simulink model "ms_project_cleaned_from_autosave"  (R2020b)
settings: Solver=VariableStepAuto  StartTime=0.0  StopTime=2  RelTol=1e-3
libraries: powerlib x19, simulink x7, powerlib_meascontrol x6, fillib x2, re_lib x1
settings Model: Creator=mcapuano  LastModifiedBy=mcapuano

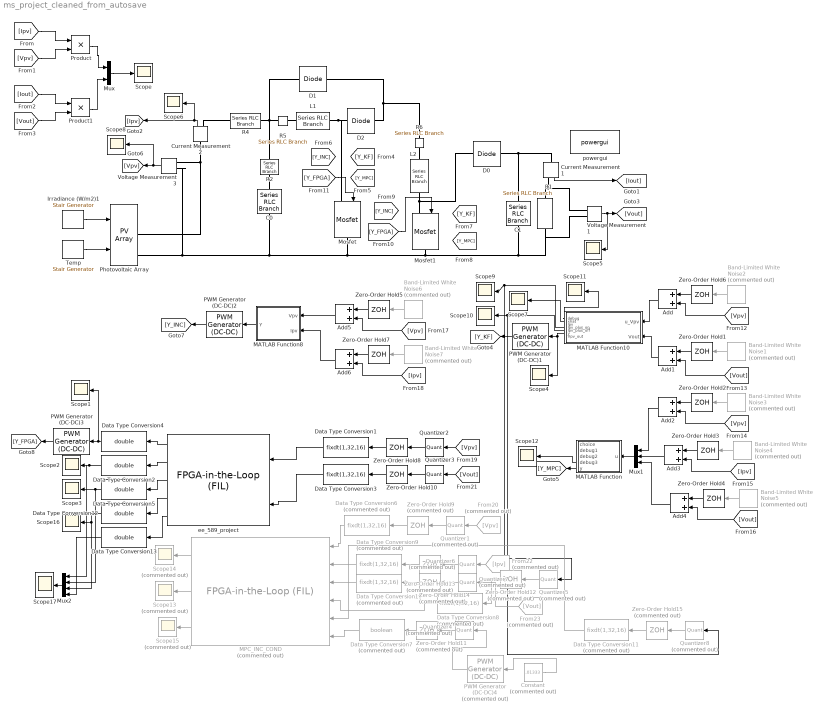
== system ms_project_cleaned_from_autosave ==
  " Temp" : powerlib_meascontrol/Pulse & Signal Generators/Stair Generator  t=[0 .5 1 1.5]  e=[25 25 35 45]  Ts=15e-6
  Add{,1..6} (7 alike) : Sum
  Band-Limited White Noise{1..7} (7 alike) : simulink/Sources/Band-Limited White Noise  Commented=on  Cov=[.00001]  Ts=15e-6  seed=[23341]
  C0 : powerlib/Elements/Series RLC Branch  LConnTagsString=__new0  RConnTagsString=__new0  BranchType=C  Resistance=1e-4  Inductance=200e-6  SetiL0=off  InitialCurrent=0  Capacitance=260e-6  Setx0=on  InitialVoltage=0  Measurements=None
  C1 : powerlib/Elements/Series RLC Branch  LConnTagsString=__new0  RConnTagsString=__new0  BranchType=C  Resistance=1e-4  Inductance=200e-6  SetiL0=off  InitialCurrent=0  Capacitance=260e-6  Setx0=on  InitialVoltage=0  Measurements=None
  Constant : Constant  Commented=on  Value=.01333
  Current Measurement1 : powerlib/Measurements/Current Measurement  PhasorSimulation=off  OutputType=Complex  PSBequivalent=0
  Current Measurement2 : powerlib/Measurements/Current Measurement  PhasorSimulation=off  OutputType=Complex  PSBequivalent=0
  D0 : powerlib/Power Electronics/Diode  Ron=1e-3  Lon=0  Vf=0  IC=0  UseSnubber=off  Rs=inf  Cs=inf  Measurements=off
  D1 : powerlib/Power Electronics/Diode  Ron=1e-3  Lon=0  Vf=0  IC=0  UseSnubber=off  Rs=inf  Cs=inf  Measurements=off
  D2 : powerlib/Power Electronics/Diode  Ron=1e-3  Lon=0  Vf=0  IC=0  UseSnubber=off  Rs=inf  Cs=inf  Measurements=off
  Data Type Conversion1 : DataTypeConversion  OutDataTypeStr=fixdt(1,32,16)
  Data Type Conversion{6,8..11} (5 alike) : DataTypeConversion  Commented=on  OutDataTypeStr=fixdt(1,32,16)
  Data Type Conversion{2,4..5,12..13} (5 alike) : DataTypeConversion  OutDataTypeStr=double
  Data Type Conversion3 : DataTypeConversion  OutDataTypeStr=fixdt(1,32,16)
  Data Type Conversion7 : DataTypeConversion  Commented=on  OutDataTypeStr=boolean
  From20 : From  Commented=on  GotoTag=Vpv
  From22 : From  Commented=on  GotoTag=Ipv
  From23 : From  Commented=on  GotoTag=Vout
  Irradiance (W/m2)1 : powerlib_meascontrol/Pulse & Signal Generators/Stair Generator  t=[0 .5]  e=[800 1000]  Ts=15e-6
  L1 : powerlib/Elements/Series RLC Branch  LConnTagsString=__new0  RConnTagsString=__new0  BranchType=L  Resistance=1e-4  Inductance=3e-3  SetiL0=on  InitialCurrent=0  Capacitance=30e-6  Setx0=off  InitialVoltage=150  Measurements=None
  L2 : powerlib/Elements/Series RLC Branch  LConnTagsString=__new0  RConnTagsString=__new0  BranchType=L  Resistance=1e-4  Inductance=3e-3  SetiL0=on  InitialCurrent=0  Capacitance=30e-6  Setx0=off  InitialVoltage=150  Measurements=None
  MATLAB Function : MATLAB Function  TreatAsAtomicUnit=on  SystemSampleTime=15e-6
  MATLAB Function10 : MATLAB Function  TreatAsAtomicUnit=on  SystemSampleTime=15e-6
  MATLAB Function8 : MATLAB Function  TreatAsAtomicUnit=on  SystemSampleTime=15e-6
  MPC_INC_COND : fillib/FPGA-in-the-Loop (FIL)  Commented=on  ForceInterfaceUpdate=0.67874
      settings: SourceProductBaseCode=ES,HD
  Mosfet : powerlib/Power Electronics/Mosfet  Ron=1e-3  Lon=0  Rd=1e-3  Vfd=0  IC=0  Rs=1e6  Cs=inf  Measurements=off
  Mosfet1 : powerlib/Power Electronics/Mosfet  Ron=1e-3  Lon=0  Rd=1e-3  Vfd=0  IC=0  Rs=1e6  Cs=inf  Measurements=off
  Mux : Mux  Inputs=2
  Mux1 : Mux  Inputs=3
  Mux2 : Mux
  PWM Generator (DC-DC)1 : powerlib_meascontrol/Pulse & Signal Generators/PWM Generator (DC-DC)  Fsw=66.67e3  Ts=0
  PWM Generator (DC-DC)2 : powerlib_meascontrol/Pulse & Signal Generators/PWM Generator (DC-DC)  Fsw=66.67e3  Ts=0
  PWM Generator (DC-DC)3 : powerlib_meascontrol/Pulse & Signal Generators/PWM Generator (DC-DC)  Fsw=66.67e3  Ts=0
  PWM Generator (DC-DC)4 : powerlib_meascontrol/Pulse & Signal Generators/PWM Generator (DC-DC)  Commented=on  Fsw=66.67e3  Ts=0
  Photovoltaic Array : re_lib/Solar/PV Array  Npar=1  Nser=1  PlotType=array @ 25 deg.C & specified irradiances  S_vec=[600 800 1000 1200]  Temp_C_vec=[25 50 75 100]  ModuleName=Kyocera Solar KC200GT  PlotWhenSelected=off  Pm=200.143  Ncell=54  Voc=32.9  Isc=8.21  Vm=26.3  Im=7.61  beta_Voc_pc=-0.355  alpha_Isc_pc=0.06  beta_Voc=-0.11679  alpha_Isc=0.004926  IL=8.2288  I0=2.3234e-10  nI=0.97734  Rsh=150.6844  Rs=0.34484  RobustModel=off  RobustCellTemperature=313.3991  BAL=on  Tc=1e-6  Tfilter=5e-5
      settings: AttributesFormatString=|
      | %<ModuleName>
      | %<Nser>-module string
      | %<Npar> parallel strings
  Product : Product
  Product1 : Product
  Quantizer{1,4..8} (6 alike) : Quantizer  Commented=on  QuantizationInterval=15e-6
  Quantizer2 : Quantizer  QuantizationInterval=15e-6
  Quantizer3 : Quantizer  QuantizationInterval=15e-6
  R1 : powerlib/Elements/Series RLC Branch  LConnTagsString=__new0  RConnTagsString=__new0  BranchType=R  Resistance=100  Inductance=200e-6  SetiL0=off  InitialCurrent=0  Capacitance=400e-6  Setx0=off  InitialVoltage=0  Measurements=None
  R2 : powerlib/Elements/Series RLC Branch  LConnTagsString=__new0  RConnTagsString=__new0  BranchType=R  Resistance=.01  Inductance=200e-6  SetiL0=off  InitialCurrent=0  Capacitance=400e-6  Setx0=off  InitialVoltage=0  Measurements=None
  R4 : powerlib/Elements/Series RLC Branch  LConnTagsString=__new0  RConnTagsString=__new0  BranchType=R  Resistance=1  Inductance=200e-6  SetiL0=off  InitialCurrent=0  Capacitance=400e-6  Setx0=off  InitialVoltage=0  Measurements=None
  R5 : powerlib/Elements/Series RLC Branch  LConnTagsString=__new0  RConnTagsString=__new0  BranchType=R  Resistance=1  Inductance=200e-6  SetiL0=off  InitialCurrent=0  Capacitance=400e-6  Setx0=off  InitialVoltage=0  Measurements=None
  R6 : powerlib/Elements/Series RLC Branch  LConnTagsString=__new0  RConnTagsString=__new0  BranchType=R  Resistance=1  Inductance=200e-6  SetiL0=off  InitialCurrent=0  Capacitance=400e-6  Setx0=off  InitialVoltage=0  Measurements=None
  Scope{,1..12,16..17} (15 alike) : Scope
  Scope13 : Scope  Commented=on
  Scope14 : Scope  Commented=on
  Scope15 : Scope  Commented=on
  Voltage Measurement1 : powerlib/Measurements/Voltage Measurement  PhasorSimulation=off  OutputType=Complex  PSBequivalent=0
  Voltage Measurement3 : powerlib/Measurements/Voltage Measurement  PhasorSimulation=off  OutputType=Complex  PSBequivalent=0
  Zero-Order Hold{1..7} (7 alike) : ZeroOrderHold  SampleTime=15e-6
  Zero-Order Hold10 : ZeroOrderHold  SampleTime=200e-9
  Zero-Order Hold{9,11..15} (6 alike) : ZeroOrderHold  Commented=on  SampleTime=200e-9
  Zero-Order Hold8 : ZeroOrderHold  SampleTime=200e-9
  ee_589_project : fillib/FPGA-in-the-Loop (FIL)  ForceInterfaceUpdate=0.046171
      settings: SourceProductBaseCode=ES,HD
  powergui : powerlib/powergui  Priority=1  SimulationMode=Continuous  SampleTime=50e-6  frequency=60  Iterations=50  frequencyindice=0  Pbase=100e6  ErrMax=1e-4  UnitsV=kV  UnitsW=MW  buscounter=0  FunctionMessages=off  echomessages=off  EnableUseOfTLC=off  CurrentSourceSwitches=off  DisableSnubberDevices=off  DisableRonSwitches=off  DisableVfSwitches=off  DisplayEquations=off  AutomaticDiscreteSolvers=off  SolverType=Tustin/Backward Euler (TBE)  Interpol=off  ExternalGateDelay=off  methode=off  Ts=100  x0status=blocks  SPID=on  SwTol=0  HookPort=off  NonlinearTolerance=1e-4  nMaxIteration=100  ContinueOnMaxIteration=off  RestoreLinks=warning  ResistiveCurrentMeasurement=off  Frange=[0:2:500]  Ylog=off  Xlog=on  ShowGrid=off  save=off  variable=ZData  structure=0  ZoomFFT=off  StartTime=0.0  cycles=1  DisplayStyle=1  fundamental=60  FreqAxis=off  MaxFrequency=1000  frequencyindicesteady=1  RmsSteady=1  display=off
  wires:
  Irradiance (W/m2)1/1 -> Photovoltaic Array/1
  " Temp"/1 -> Photovoltaic Array/2
  Voltage Measurement3/1 -> Scope8/1, [Vpv]
  Current Measurement2/1 -> Scope6/1, [Ipv]
  Voltage Measurement1/1 -> Scope5/1, [Vout]
  Current Measurement1/1 -> [Iout]
  [Ipv] -> Product/1
  [Vpv] -> Product/2
  Mux/1 -> Scope/1
  Product/1 -> Mux/1
  [Vout] -> Product1/2
  [Iout] -> Product1/1
  Product1/1 -> Mux/2
  Band-Limited White Noise2/1 -> Zero-Order Hold6/1
  MATLAB Function10/6(y) -> Scope4/1, PWM Generator (DC-DC)1/1
  PWM Generator (DC-DC)1/1 -> [Y_KF]
  Add/1 -> MATLAB Function10/1(u_Vpv)
  Zero-Order Hold6/1 -> Add/1
  Band-Limited White Noise1/1 -> Zero-Order Hold1/1
  Zero-Order Hold1/1 -> Add1/1
  Add1/1 -> MATLAB Function10/2(Vout)
  [Vpv] -> Add/2
  [Vout] -> Add1/2
  MATLAB Function/5(y) -> [Y_MPC]
  Mux1/1 -> MATLAB Function/1(u)
  [Vpv] -> Add2/2
  Band-Limited White Noise3/1 -> Zero-Order Hold2/1
  Zero-Order Hold2/1 -> Add2/1
  Add2/1 -> Mux1/1
  [Ipv] -> Add3/2
  Band-Limited White Noise4/1 -> Zero-Order Hold3/1
  Zero-Order Hold3/1 -> Add3/1
  Add3/1 -> Mux1/2
  Band-Limited White Noise5/1 -> Zero-Order Hold4/1
  [Vout] -> Add4/2
  Zero-Order Hold4/1 -> Add4/1
  Add4/1 -> Mux1/3
  [Vpv] -> Add5/2
  Band-Limited White Noise7/1 -> Zero-Order Hold7/1
  Band-Limited White Noise6/1 -> Zero-Order Hold5/1
  [Ipv] -> Add6/2
  Zero-Order Hold7/1 -> Add6/1
  Zero-Order Hold5/1 -> Add5/1
  Add5/1 -> MATLAB Function8/1(Vpv)
  Add6/1 -> MATLAB Function8/2(Ipv)
  [Vpv] -> Quantizer2/1
  Quantizer2/1 -> Zero-Order Hold8/1
  Zero-Order Hold8/1 -> Data Type Conversion1/1
  Quantizer3/1 -> Zero-Order Hold10/1
  Zero-Order Hold10/1 -> Data Type Conversion3/1
  Data Type Conversion3/1 -> ee_589_project/2
  [Vout] -> Quantizer3/1
  ee_589_project/1 -> Data Type Conversion4/1
  PWM Generator (DC-DC)2/1 -> [Y_INC]
  MATLAB Function8/1(Y) -> PWM Generator (DC-DC)2/1
  PWM Generator (DC-DC)3/1 -> [Y_FPGA]
  Data Type Conversion4/1 -> Scope1/1, PWM Generator (DC-DC)3/1
  Data Type Conversion1/1 -> ee_589_project/1
  ee_589_project/2 -> Data Type Conversion2/1
  ee_589_project/3 -> Data Type Conversion5/1
  Data Type Conversion2/1 -> Mux2/1, Scope2/1
  Data Type Conversion5/1 -> Mux2/2, Scope3/1
  MATLAB Function10/2(xhat) -> Scope7/1
  MATLAB Function10/4(Ipv_plus_on) -> Quantizer5/1, Scope9/1
  MATLAB Function10/5(Ipv_plus_off) -> Quantizer8/1, Scope10/1
  MATLAB Function10/1(debug) -> Scope11/1
  MATLAB Function/4(debug3) -> Scope12/1
  Data Type Conversion6/1 -> MPC_INC_COND/1
  Zero-Order Hold9/1 -> Data Type Conversion6/1
  Quantizer1/1 -> Zero-Order Hold9/1
  From20/1 -> Quantizer1/1
  Zero-Order Hold12/1 -> Data Type Conversion8/1
  Quantizer5/1 -> Zero-Order Hold12/1
  Data Type Conversion8/1 -> MPC_INC_COND/4
  Zero-Order Hold13/1 -> Data Type Conversion9/1
  Quantizer6/1 -> Zero-Order Hold13/1
  Data Type Conversion9/1 -> MPC_INC_COND/2
  Zero-Order Hold14/1 -> Data Type Conversion10/1
  Quantizer7/1 -> Zero-Order Hold14/1
  Data Type Conversion10/1 -> MPC_INC_COND/3
  From22/1 -> Quantizer6/1
  From23/1 -> Quantizer7/1
  MPC_INC_COND/3 -> Scope15/1
  MPC_INC_COND/1 -> Scope14/1
  MPC_INC_COND/2 -> Scope13/1
  Data Type Conversion11/1 -> MPC_INC_COND/5
  Zero-Order Hold15/1 -> Data Type Conversion11/1
  Quantizer8/1 -> Zero-Order Hold15/1
  Data Type Conversion7/1 -> MPC_INC_COND/6
  Zero-Order Hold11/1 -> Data Type Conversion7/1
  Quantizer4/1 -> Zero-Order Hold11/1
  PWM Generator (DC-DC)4/1 -> Quantizer4/1
  Constant/1 -> PWM Generator (DC-DC)4/1
  [Y_FPGA] -> Mosfet/1
  [Y_FPGA] -> Mosfet1/1
  ee_589_project/4 -> Data Type Conversion12/1
  ee_589_project/5 -> Data Type Conversion13/1
  Data Type Conversion12/1 -> Mux2/3, Scope16/1
  Mux2/1 -> Scope17/1
  Data Type Conversion13/1 -> Mux2/4
  connections:
  Voltage Measurement3/LConn1 -- Current Measurement2/LConn1 -- Photovoltaic Array/RConn1
  R4/LConn1 -- Current Measurement2/RConn1
  R5/LConn1 -- R4/RConn1 -- R2/LConn1 -- D1/LConn1
  R5/RConn1 -- L1/LConn1
  D2/LConn1 -- Mosfet/LConn1 -- L1/RConn1
  D1/RConn1 -- R6/LConn1 -- D2/RConn1
  L2/LConn1 -- R6/RConn1
  Mosfet1/LConn1 -- D0/LConn1 -- L2/RConn1
  C0/LConn1 -- R2/RConn1
  C0/RConn1 -- Voltage Measurement3/LConn2 -- Photovoltaic Array/RConn2 -- Voltage Measurement1/LConn2 -- R1/RConn1 -- C1/RConn1 -- Mosfet1/RConn1 -- Mosfet/RConn1
  C1/LConn1 -- Current Measurement1/LConn1 -- D0/RConn1
  Current Measurement1/RConn1 -- Voltage Measurement1/LConn1 -- R1/LConn1

== matlab function ms_project_cleaned_from_autosave/MATLAB Function ==
  settings: updateMethod=DISCRETE
  data: choice output; debug1 output; debug2 output; debug3 output; u input; y output
function [choice, debug1, debug2,debug3, y]= fcn(u)
Vpv=u(1);
Ipv=u(2);
Vout=u(3);

%This module contains the MPC-MPPT Control Algorithm

%The MPC module follows the flow chart of Fig. 8 in Referenced Research Paper

%This MATLAB fn block's settings have been changed to have a sampling rate
%of 15uS instead of being continous sample mode


%prevent crazy simulation transients from breaking the algorithm:
if (Ipv > 10)
    Ipv = 1;
end

persistent Vpv_t_1; %previous Vpv Sample
if isempty(Vpv_t_1)
    Vpv_t_1 = 0;
end
persistent Ipv_t_1; %previous Ipv Sample
if isempty(Ipv_t_1)
    Ipv_t_1 = 0;
end
persistent Dpv_t_1; % Iref (output) value from what is now 2 timesteps ago
if isempty(Dpv_t_1)
    Dpv_t_1 = 0;
end
persistent Dpv;  %Previous / Most recent Iref (output) Calc
if isempty(Dpv)
    Dpv = 0;
end

Ts = 15e-6; %sample rate
L = 3e-3; %inductance

Power = Vpv * Ipv;
delta_P = Power - (Vpv_t_1 * Ipv_t_1);
delta_V = Vpv - Vpv_t_1;
delta_I = Ipv - Ipv_t_1;
delta_D = Dpv - Dpv_t_1;


%fixed vs adaptive
S = .001;
M = 10;
Z =.001;%delta_P/delta_V * exp(-M*Dpv); %.0005; %fixed 
%Z = scale_factor_C * abs(delta_I * delta_D); %adaptive

% custom adaptive to fix issues with no change causing 0 step size
 %adapZ = scale_factor_C * abs(delta_I * delta_D);
% if(adapZ > .1)
%     Z = .1;
% elseif(adapZ > .001)
%     Z = adapZ;
% else
%     Z = .001;
% end


Ipred_1 = Ipv + 2*(Ts/L) * Vpv; %MPC prediction for switch = 1
Ipred_0 = Ipv + (Ts/(2*L)* (Vpv - Vout)); %MPC prediction for switch = 0 

if delta_V == 0 %Inc. Cond. Algo to determin Iref
    if delta_I == 0 
        Iref = Dpv; choice = 0;
    else
        if delta_I > 0
            Iref = Dpv - Z; choice = 1;
        else
            Iref = Dpv + Z; choice = 2;
        end
    end
else
    if (Ipv + (delta_I/delta_V) * Vpv) == 0
        Iref = Dpv; choice = 3;
    else
        if (Ipv + (delta_I/delta_V) * Vpv) > 0
            Iref = Dpv - Z; choice = 4;
        else
            Iref = Dpv + Z; choice = 5;
        end
    end
end

G1 = abs(Iref - Ipred_1); %Optimize MPC by applying Iref
G0 = abs(Iref - Ipred_0);
if G1 < G0
    y = 1;
else
    y = 0;
end

if (Iref < 0)
    Iref = .001;
end
%test = Ipv + (delta_I/delta_V) * Vpv;
test =  delta_V;
%update static variables here:
Vpv_t_1 = Vpv; %previous Vpv Sample
Ipv_t_1 = Ipv; %previous Ipv Sample
Dpv_t_1 = Dpv; % Iref (output) value from what is now 2 timesteps ago
Dpv = Iref;  %Previous / Most recent Iref (output) Calc

%debug purposes:
debug1 = Ipred_1;
debug2 = Ipred_0;
debug3 = Iref;

== matlab function ms_project_cleaned_from_autosave/MATLAB Function8 ==
  settings: updateMethod=DISCRETE
  data: Y output; Vpv input; Ipv input
function Y= fcn(Vpv, Ipv)

persistent DC;
if isempty(DC)
    DC = 0;
end

persistent Vpv_t_1;
if isempty(Vpv_t_1)
    Vpv_t_1 = 0;
end
persistent Ipv_t_1;
if isempty(Ipv_t_1)
    Ipv_t_1 = 0;
end

Delta_V = Vpv - Vpv_t_1;
Delta_I = Ipv - Ipv_t_1;

if (Delta_V == 0 && Delta_I == 0) DC = DC; 
elseif (Delta_V == 0 && Delta_I > 0) DC = DC - .0005; 
elseif (Delta_V == 0 && Delta_I < 0) DC = DC + .0005; 
elseif (Delta_V ~= 0 && Delta_I/Delta_V == -Ipv/Vpv) DC = DC; 
elseif (Delta_V ~= 0 && Delta_I/Delta_V ~= -Ipv/Vpv && Delta_I/Delta_V > -Ipv/Vpv) DC = DC - .0005; 
elseif (Delta_V ~= 0 && Delta_I/Delta_V ~= -Ipv/Vpv && Delta_I/Delta_V < -Ipv/Vpv) DC = DC + .0005; 
end
% Z = .001;
% if Delta_V == 0 %Inc. Cond. Algo to determin DC
%     if delta_I == 0 
%         DC = DC; choice = 0;
%     else
%         if delta_I > 0
%             DC = DC - Z; choice = 1;
%         else
%             DC = DC + Z; choice = 2;
%         end
%     end
% else
%     if (Ipv + (delta_I/Delta_V) * Vpv) == 0
%         DC = DC; choice = 3;
%     else
%         if (Ipv + (delta_I/Delta_V) * Vpv) > 0
%             DC = DC - Z; choice = 4;
%         else
%             DC = DC + Z; choice = 5;
%         end
%     end
% end


if(DC < 0) DC = 0; end
if(DC > 1) DC = 1; end

Vpv_t_1 = Vpv;
Ipv_t_1 = Ipv;
Y = DC;

== matlab function ms_project_cleaned_from_autosave/MATLAB Function10 ==
  data: debug output; xhat output; u_Vpv input; Vout input; Ipv output; Ipv_plus_on output; Ipv_plus_off output; y output; Vpv_out output
function [debug, xhat, Ipv, Ipv_plus_on, Ipv_plus_off, y, Vpv_out]  = fcn(u_Vpv, Vout)
%Kalman filter design using Small Signal Model of Circuit

%The purpose of this module is to approximate Ipv and Vpv so that a sensor
%is not needed for those variables, it also functions to remove noise and
%could possibly replace the MCP module using its own predictions

%Existing Model assumes Constant Vpv with added series resistor so that
% Ipv = (Vpv - Vcpv)/Rpv
%Also assumes L1 = L2

%Existing state variables: IL1 IL2 Vo Vcpv

%define circuit parameters 


Cpv=260e-6;
Cout=260e-6;
L1=3e-3;
L2=3e-3;
Rout=100;
Rpv = 1;
RL1 = 1;
RL2 = 1;

persistent Est_Vpv;
if isempty(Est_Vpv)
    Est_Vpv = 0;
end
persistent DC;
if isempty(DC)
    DC = 1;
end
Vpv = u_Vpv;
y = Vout;
u = u_Vpv;

Ts = 15e-6;
% Continuous Time Small Signal State Space
%Aol = [0.943784461257301,-0.0559330122345799,-0.0279395312339836,5.29606701473712e-05;0.00363447688363775,0.996152021590196,-0.00131615408875196,-0.00124644633684318;0.00363447688363775,-0.00135110080726459,0.996186968308708,-0.00124644633684318;5.29606701473712e-05,-1.90030480999995e-05,0.0287831492829427,0.999405251934562];
Ac =[(-1/(Cpv*Rpv)) (-1/(Cpv)) (-DC/(Cpv)) 0 ;
    (1/(L1+L2) + L2*DC/(L1*(L1+L2)))  (-RL1/(L1+L2) -RL1*L2*DC/(L1*(L1+L2)))  (-RL2/(L1+L2) + RL2*DC/(L1+L2)) (-1/(L1+L2) + DC/(L1+L2));
    (1/(L1+L2) + L1*DC/(L2*(L1+L2)))  (-RL1/(L1+L2) + RL1*DC/(L1+L2)) (-RL2/(L1+L2)-RL2*L1*DC/(L2*(L1+L2))) (-1/(L1+L2) + DC/(L1+L2));
    0 0 (1/(Cout) - DC/(Cout)) (-1/(Rout*Cout))];
Bc = [1/(Cpv*Rpv);
    0;
    0;
    0];
 Cc = [0 0 0 1];
 
 Dc = zeros(size(Cc,1), size(Bc,2));
 
 %discretize my state space model using ZOH method
 Aol = eye(4) + Ac*Ts;
 Bol = Bc*Ts;
 Col = Cc;
 Dol = Dc;
 
 
%Bol = [0.0560566260169120;0.000105941817191590;0.000105941817191590;1.02384484238660e-06];

%Col = [0,0,0,1];

%Dol = 0;
 %Design the Observer System:
 

 %covar matricies, process q, measurement r -- must be positive numbers
 Qcov = diag(.0001*ones(1,4)); %modify the numbers to change how it filters noise
 Rcov = diag(.01*ones(1,1)); %modify the numbers to change how it filters noise
 

persistent xhat_t_1; %previous xhat Sample
if isempty(xhat_t_1)
    xhat_t_1 = [.1; .1; .1; .1];
end

persistent P_t_1;
if isempty(P_t_1)
    P_t_1 = [.1 .1 .1 .1;
            .1 .1 .1 .1;
            .1 .1 .1 .1;
            .1 .1 .1 .1];
end


%prediction stage
xhat_pred = Aol*xhat_t_1+Bol*u;
P_pred = Aol*P_t_1*transpose(Aol)+ Qcov;

%update stage
y_update = y - Col*xhat_pred;
S_update = Col*P_pred*transpose(Col) + Rcov;
K_update = P_pred*transpose(Col)*(1/S_update);
xhat_update = xhat_pred + K_update*y_update;
P_update = (eye(4) - K_update*Col)*P_pred;

Est_Vpv =  xhat_update(4)*(1-DC)/(1+DC) + .35;
 Vpv_out = Est_Vpv;

%increase DC by .01:
DC = DC + .0001;
if(DC > 1)
    DC = 1;
end
Ac =[(-1/(Cpv*Rpv)) (-1/(Cpv)) (-DC/(Cpv)) 0 ;
    (1/(L1+L2) + L2*DC/(L1*(L1+L2)))  (-RL1/(L1+L2) -RL1*L2*DC/(L1*(L1+L2)))  (-RL2/(L1+L2) + RL2*DC/(L1+L2)) (-1/(L1+L2) + DC/(L1+L2));
    (1/(L1+L2) + L1*DC/(L2*(L1+L2)))  (-RL1/(L1+L2) + RL1*DC/(L1+L2)) (-RL2/(L1+L2)-RL2*L1*DC/(L2*(L1+L2))) (-1/(L1+L2) + DC/(L1+L2));
    0 0 (1/(Cout) - DC/(Cout)) (-1/(Rout*Cout))];
Aol_increase = eye(4) + Ac*Ts;
%predict 1 timestep ahead on
xhat_plus_on = Aol_increase*xhat_update + Bol*u;
Ipv_plus_on = (u - xhat_plus_on(1))/Rpv;
%decrease DC by .01
DC = DC - 2*.0001;
if(DC < 0) 
    DC = 0; end
Ac =[(-1/(Cpv*Rpv)) (-1/(Cpv)) (-DC/(Cpv)) 0 ;
    (1/(L1+L2) + L2*DC/(L1*(L1+L2)))  (-RL1/(L1+L2) -RL1*L2*DC/(L1*(L1+L2)))  (-RL2/(L1+L2) + RL2*DC/(L1+L2)) (-1/(L1+L2) + DC/(L1+L2));
    (1/(L1+L2) + L1*DC/(L2*(L1+L2)))  (-RL1/(L1+L2) + RL1*DC/(L1+L2)) (-RL2/(L1+L2)-RL2*L1*DC/(L2*(L1+L2))) (-1/(L1+L2) + DC/(L1+L2));
    0 0 (1/(Cout) - DC/(Cout)) (-1/(Rout*Cout))];
DC = DC + .0001;
Aol_decrease = eye(4) + Ac*Ts;
%predict 1 timestep ahead off
xhat_plus_off = Aol_decrease*xhat_update + Bol*u;
Ipv_plus_off = (u - xhat_plus_off(1))/Rpv;

%update function output and variables
P_t_1 = P_update;
xhat_t_1 = xhat_update;
xhat = xhat_update;
Ipv = (u - xhat(1))/Rpv;

%%%%%%%%%%%%%%%%%%%%%%%%%%%%%%%
if (Ipv > 10)
    Ipv = 1;
end



persistent Vpv_t_1; %previous Vpv Sample
if isempty(Vpv_t_1)
    Vpv_t_1 = 0;
end
persistent Ipv_t_1; %previous Ipv Sample
if isempty(Ipv_t_1)
    Ipv_t_1 = 0;
end
persistent Dpv_t_1; % Iref (output) value from what is now 2 timesteps ago
if isempty(Dpv_t_1)
    Dpv_t_1 = 0;
end
persistent Dpv;  %Previous / Most recent Iref (output) Calc
if isempty(Dpv)
    Dpv = 0;
end

Ts = 15e-6; %sample rate
L = 3e-3; %inductance


delta_V = Vpv - Vpv_t_1;
delta_I = Ipv - Ipv_t_1;
delta_D = Dpv - Dpv_t_1;


%fixed vs adaptive
scale_factor_C = 10; %increase for larger output increments/swings
 Z =.001; %fixed 
%Z = scale_factor_C * abs(delta_I * delta_D); %adaptive

% custom adaptive to fix issues with no change causing 0 step size
 adapZ = scale_factor_C * abs(delta_I * delta_D);
% if(adapZ > .1)
%     Z = .1;
% elseif(adapZ > .001)
%     Z = adapZ;
% else
%     Z = .001;
% end

Ipred_1 = Ipv_plus_on;
Ipred_0 = Ipv_plus_off;
%Ipred_1 = Ipv + 2*(Ts/L) * Vpv; %MPC prediction for switch = 1
%Ipred_0 = Ipv + (Ts/(2*L)* (Vpv - Vout)); %MPC prediction for switch = 0 

if delta_V == 0 %Inc. Cond. Algo to determine Iref
    if delta_I == 0 
        Iref = Dpv; choice = 0;
    else
        if delta_I > 0
            Iref = Dpv - Z; choice = 1;
        else
            Iref = Dpv + Z; choice = 2;
        end
    end
else
    if (Ipv + (delta_I/delta_V) * Vpv) == 0
        Iref = Dpv; choice = 3;
    else
        if (Ipv + (delta_I/delta_V) * Vpv) > 0
            Iref = Dpv - Z; choice = 4;
        else
            Iref = Dpv + Z; choice = 5;
        end
    end
end

G1 = abs(Iref - Ipred_1); %Optimize MPC by applying Iref
G0 = abs(Iref - Ipred_0);
if G1 < G0
    DC = DC + .0001;
else
    DC = DC - .0001;
end

if (DC < 0)
    DC = 0;
end
if (DC > 1)
    DC = 1;
end

if (Iref < 0)
    Iref = .001;
end
%test = Ipv + (delta_I/delta_V) * Vpv;
test =  delta_V;
%update static variables here:
Vpv_t_1 = Vpv; %previous Vpv Sample
Ipv_t_1 = Ipv; %previous Ipv Sample
Dpv_t_1 = Dpv; % Iref (output) value from what is now 2 timesteps ago
Dpv = Iref;  %Previous / Most recent Iref (output) Calc

y = DC;

%debug purposes:
debug = Iref;
